simulink model "oneforall_sim"  (R2017b)
settings: Solver=ode4  StartTime=0.0  StopTime=100  FixedStep=0.1  RelTol=1e-3
values from neighbouring files (symbols this model uses):
  A = [-.0213 0 0; 0.0006 -0.005 0;0 -0.00038 -0.0023]    [kalman.m]    (also in med_utf8.m = [A11 A12 ; A21 A22]; oneforall.m = [A11 A12 ; A21 A22])
  B = [8.9362;0;0]    [kalman.m]    (also in med_utf8.m = [0;1/m]; oneforall.m = [0;1/m])
  C = eye(3)    [kalman.m]    (also in med_utf8.m = [1 0]; oneforall.m = [1 0])
undefined symbols (not defined in the file or in its folder): Kopt
settings Model: Creator=lencs  LastModifiedBy=lencs

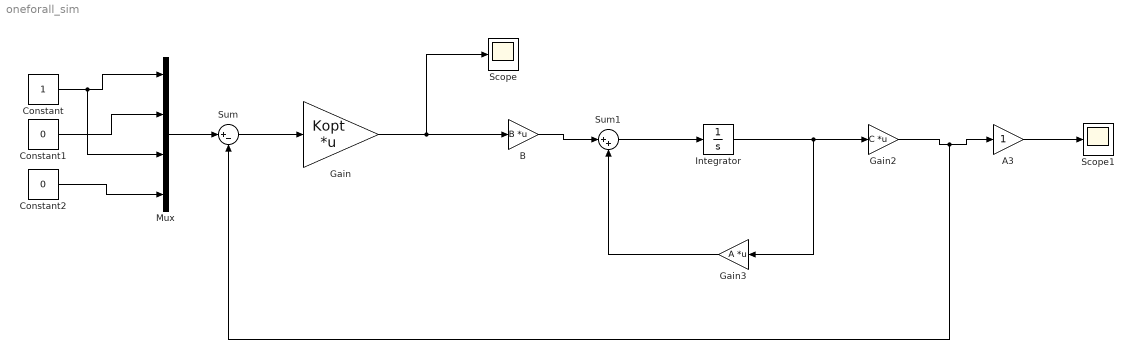
== system oneforall_sim ==
  "A3 " : Gain
  B : Gain  Gain=B  Multiplication=Matrix(K*u)
  Constant : Constant
  Constant1 : Constant  Value=0
  Constant2 : Constant  Value=0
  Gain : Gain  Gain=Kopt  Multiplication=Matrix(K*u)
  Gain2 : Gain  Gain=C  Multiplication=Matrix(K*u)
  Gain3 : Gain  Gain=A  Multiplication=Matrix(K*u) (u vector)
  Integrator : Integrator  InitialCondition=[0.1;0;0;0]
  Mux : Mux
  Scope : Scope
  Scope1 : Scope
  Sum : Sum  Inputs=|+-
  Sum1 : Sum  Inputs=|++
  wires:
  Gain2/1 -> Sum/2, "A3 "/1
  Mux/1 -> Sum/1
  Integrator/1 -> Gain3/1, Gain2/1
  Constant/1 -> Mux/3, Mux/1
  Sum/1 -> Gain/1
  Constant1/1 -> Mux/2
  Gain3/1 -> Sum1/2
  Constant2/1 -> Mux/4
  "A3 "/1 -> Scope1/1
  Sum1/1 -> Integrator/1
  Gain/1 -> Scope/1, B/1
  B/1 -> Sum1/1
